simulink model "reg_od_stanu"  (R2014b)
settings: Solver=ode45  StartTime=0.0  StopTime=10.0  RelTol=1e-3
values from neighbouring files (symbols this model uses):
  K = place(A2, B2, [z1 z2 z3])    [zad_6.m]
  x0 = [ -1; -2; -3 ]    [zad_6.m]
undefined symbols (not defined in the file or in its folder): A2, B2, Tp
settings Model: Creator=Konrad  LastModifiedBy=Konrad

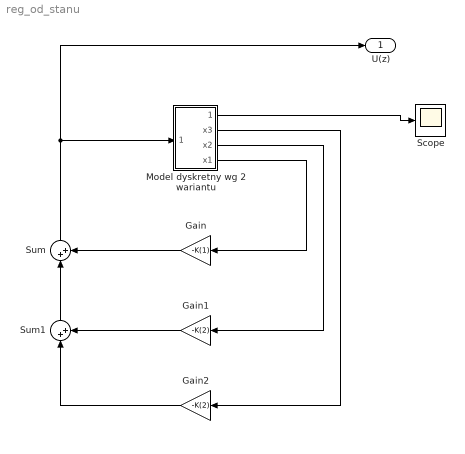
== system reg_od_stanu ==
  Gain : Gain  Gain=-K(1)
  Gain1 : Gain  Gain=-K(2)
  Gain2 : Gain  Gain=-K(2)
  Model dyskretny wg 2 wariantu : Subsystem
  Scope : Scope
  Sum : Sum  Inputs=|++
  Sum1 : Sum  Inputs=|++
  U(z) : Outport
  wires:
  Sum/1 -> U(z)/1, Model dyskretny wg 2 wariantu/1(U(z))
  Model dyskretny wg 2 wariantu/4(x1) -> Gain/1
  Model dyskretny wg 2 wariantu/3(x2) -> Gain1/1
  Model dyskretny wg 2 wariantu/2(x3) -> Gain2/1
  Gain/1 -> Sum/2
  Gain1/1 -> Sum1/2
  Gain2/1 -> Sum1/1
  Sum1/1 -> Sum/1
  Model dyskretny wg 2 wariantu/1(Y(z)) -> Scope/1

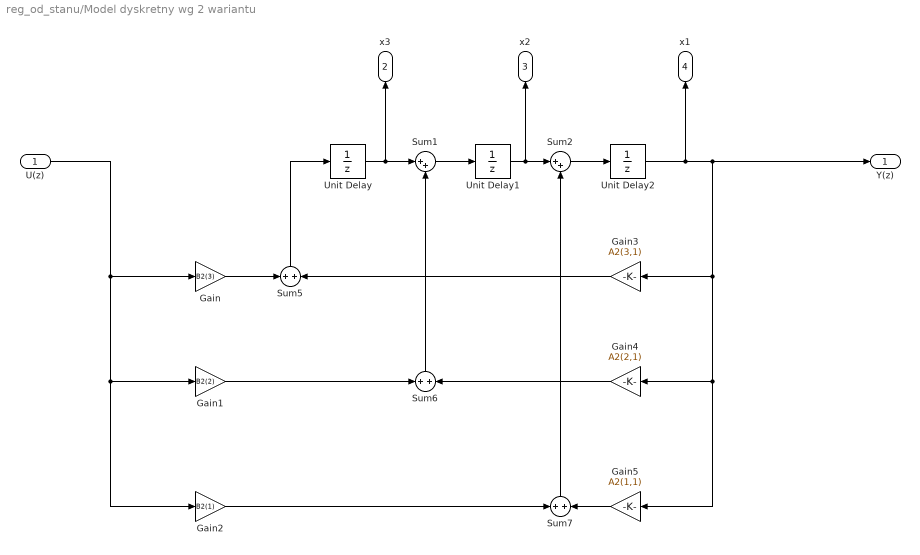
== system reg_od_stanu/Model dyskretny wg 2 wariantu ==
  U(z) : Inport
  Gain : Gain  Gain=B2(3)
  Gain1 : Gain  Gain=B2(2)
  Gain2 : Gain  Gain=B2(1)
  Gain3 : Gain  Gain=A2(3,1)
  Gain4 : Gain  Gain=A2(2,1)
  Gain5 : Gain  Gain=A2(1,1)
  Sum1 : Sum  Inputs=|++
  Sum2 : Sum  Inputs=|++
  Sum5 : Sum  Inputs=+|+
  Sum6 : Sum  Inputs=+|+
  Sum7 : Sum  Inputs=+|+
  Unit Delay : UnitDelay  InitialCondition=x0(3)  SampleTime=Tp
  Unit Delay1 : UnitDelay  InitialCondition=x0(2)  SampleTime=Tp
  Unit Delay2 : UnitDelay  InitialCondition=x0(1)  SampleTime=Tp
  Y(z) : Outport
  x3 : Outport  Port=2
  x2 : Outport  Port=3
  x1 : Outport  Port=4
  wires:
  Sum1/1 -> Unit Delay1/1
  Unit Delay1/1 -> x2/1, Sum2/1
  Sum2/1 -> Unit Delay2/1
  Unit Delay/1 -> x3/1, Sum1/1
  Gain1/1 -> Sum6/1
  Gain4/1 -> Sum6/2
  Unit Delay2/1 -> x1/1, Y(z)/1, Gain3/1, Gain4/1, Gain5/1
  Gain3/1 -> Sum5/2
  Gain/1 -> Sum5/1
  Gain5/1 -> Sum7/2
  Sum7/1 -> Sum2/2
  Sum5/1 -> Unit Delay/1
  Gain2/1 -> Sum7/1
  Sum6/1 -> Sum1/2
  U(z)/1 -> Gain/1, Gain1/1, Gain2/1
